simulink model "untitled2"  (R2024a)
settings: Solver=VariableStepAuto  StartTime=0.0  StopTime=10.0  RelTol=1e-3
settings Model: Creator=Perij  LastModifiedBy=Perij

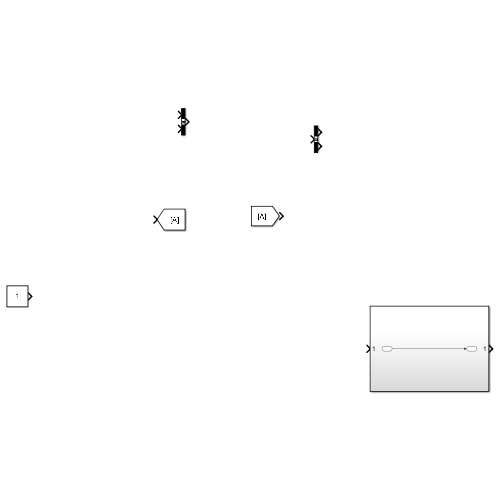
[thumbnail: Simulink's stored preview of the top-level diagram]
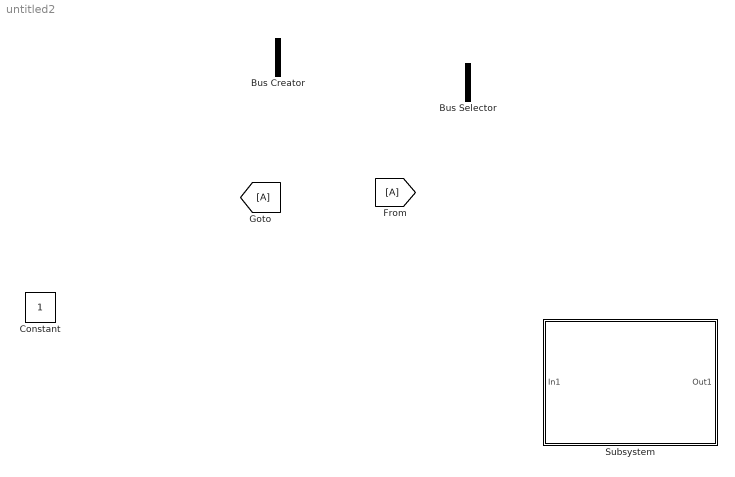
== system untitled2 ==
  Bus Creator : BusCreator  Inputs=2
  Bus Selector : BusSelector  OutputSignals=signal1,signal2
  Constant : Constant
  From : From
  Goto : Goto
  Subsystem : Subsystem

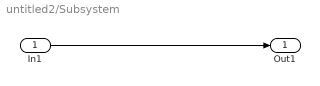
== system untitled2/Subsystem ==
  In1 : Inport
  Out1 : Outport
  wires:
  In1/1 -> Out1/1
